simulink model "PID_Test"  (R2014b)
settings: Solver=ode14x  StartTime=0.0  StopTime=inf  FixedStep=0.2  RelTol=1e-3
undefined symbols (not defined in the file or in its folder): IsPositionTracked, IsSkeletonTracked, JointDepthIndices, JointImageIndices, JointTrackingState, JointWorldCoordinates, none, PositionDepthIndices, PositionImageIndices, PositionWorldCoordinates, SegmentationData, SkeletonTrackingID, videoinput
libraries: simulink x7, arduino_io_lib x2, visionsinks x2, visionstatistics x1, visiontextngfix x1, imaqlib x1, visiongeotforms x1
settings Model: Creator=mtsou_000  LastModifiedBy=mtsou_000

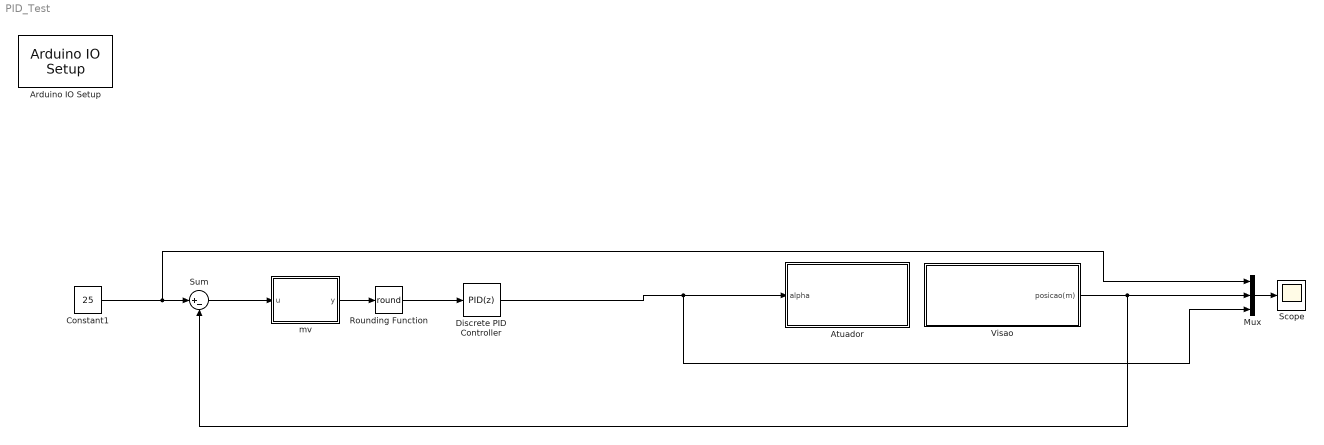
== system PID_Test ==
  Arduino IO Setup : arduino_io_lib/Arduino IO Setup  Priority=3  arduinoVar=Temporary arduino variable: Arduino1  workspaceVarName=a  comPort=COM8
  "Atuador " : Subsystem
  Constant1 : Constant  Value=25
  Discrete PID Controller : simulink/Continuous/PID Controller  Controller=PID  TimeDomain=Discrete-time  SampleTime=0.2  IntegratorMethod=Forward Euler  FilterMethod=Forward Euler  Form=Parallel  P=0.4  I=0.1  D=0.7  N=100  InitialConditionSource=internal  InitialConditionForIntegrator=0  InitialConditionForFilter=0  ExternalReset=none  LimitOutput=on  UpperSaturationLimit=30  LowerSaturationLimit=-30  LinearizeAsGain=off  AntiWindupMode=none  Kb=1  TrackingMode=off  Kt=1  PParamMin=[]  PParamMax=[]  IParamMin=[]  IParamMax=[]  DParamMin=[]  DParamMax=[]  NParamMin=[]  NParamMax=[]  KbParamMin=[]  KbParamMax=[]  KtParamMin=[]  KtParamMax=[]  POutMin=[]  POutMax=[]  IOutMin=[]  IOutMax=[]  DOutMin=[]  DOutMax=[]  NOutMin=[]  NOutMax=[]  KbOutMin=[]  KbOutMax=[]  KtOutMin=[]  KtOutMax=[]  IntegratorOutMin=[]  IntegratorOutMax=[]  FilterOutMin=[]  FilterOutMax=[]  SumOutMin=[]  SumOutMax=[]  SumI1OutMin=[]  SumI1OutMax=[]  SumI2OutMin=[]  SumI2OutMax=[]  SumI3OutMin=[]  SumI3OutMax=[]  SumDOutMin=[]  SumDOutMax=[]  SaturationOutMin=[]  SaturationOutMax=[]  IntegratorContinuousStateAttributes=''  IntegratorStateMustResolveToSignalObject=off  IntegratorRTWStateStorageClass=Auto  FilterContinuousStateAttributes=''  FilterStateMustResolveToSignalObject=off  FilterRTWStateStorageClass=Auto  DifferentiatorICPrevScaledInput=0  DifferentiatorOutMin=[]  DifferentiatorOutMax=[]  UseFilter=off
  Mux : Mux  Inputs=3
  Rounding Function : Rounding  Operator=round
  Scope : Scope
      settings: TickLabels=on  TimeRange=10  YMax=30
  Sum : Sum  Inputs=|+-
  Visao : Subsystem
  "mv " : MATLAB Function  TreatAsAtomicUnit=on
  wires:
  Sum/1 -> "mv "/1(u)
  "mv "/1(y) -> Rounding Function/1
  Mux/1 -> Scope/1
  Visao/1(posicao(m)) -> Mux/2, Sum/2
  Constant1/1 -> Mux/1, Sum/1
  Rounding Function/1 -> Discrete PID Controller/1
  Discrete PID Controller/1 -> Mux/3, "Atuador "/1(alpha)

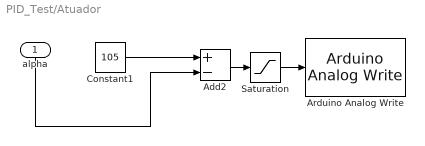
== system PID_Test/Atuador  ==
  alpha : Inport
  Add2 : Sum  Inputs=+-
  Arduino Analog Write : arduino_io_lib/Arduino Analog Write  arduinoVar=Temporary arduino variable: Arduino1  arduinoPin=3  T=0.2
  Constant1 : Constant  Value=105
  Saturation : Saturate  UpperLimit=120  LowerLimit=60
  wires:
  Add2/1 -> Saturation/1
  alpha/1 -> Add2/2
  Saturation/1 -> Arduino Analog Write/1
  Constant1/1 -> Add2/1

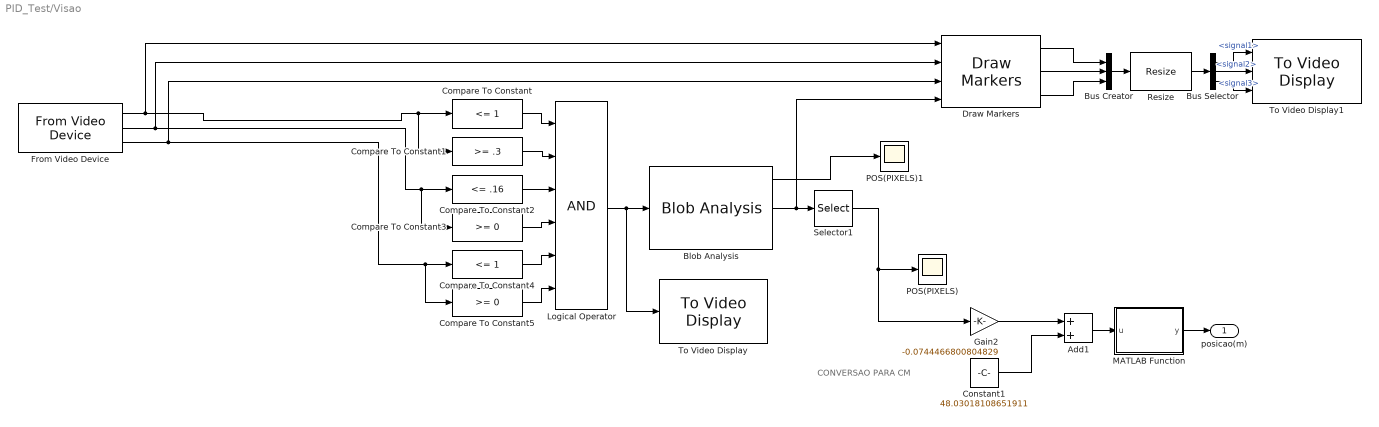
== system PID_Test/Visao ==
  note: CONVERSAO PARA CM
  Add1 : Sum
  Blob Analysis : visionstatistics/Blob Analysis  Tag=vipblks_row_conv  area=on  centroid=on  bBox=off  majorAxis=off  minorAxis=off  angle=off  eccentricity=off  equivDiameterSq=on  extent=off  perimeter=off  maxBlobs=1  warnIfNumBlobsExceeded=off  isCount=off  useMinArea=on  minArea=400  useMaxArea=off  maxArea=2200  excludeBorderBlob=off  outDT=double  isOutVarDim=off  isFill=on  fillValues=-1  conn=8  isLabel=off  outputMode=Binary point scaling  outputWordLength=32  outputFracLength=16  firstCoeffMode=Binary point scaling  firstCoeffWordLength=16  firstCoeffFracLength=14  secondCoeffMode=Binary point scaling  secondCoeffWordLength=32  secondCoeffFracLength=16  accumMode=Binary point scaling  accumWordLength=32  accumFracLength=0  prodOutputMode=Binary point scaling  prodOutputWordLength=32  prodOutputFracLength=16  roundingMode=Floor  overflowMode=off
  Bus Creator : BusCreator  Inputs=3
  Bus Selector : BusSelector
  Compare To Constant : simulink/Logic and Bit Operations/Compare To Constant  relop=<=  const=1  OutDataTypeStr=boolean
  Compare To Constant1 : simulink/Logic and Bit Operations/Compare To Constant  relop=>=  const=.3  OutDataTypeStr=boolean
  Compare To Constant2 : simulink/Logic and Bit Operations/Compare To Constant  relop=<=  const=.16  OutDataTypeStr=boolean
  Compare To Constant3 : simulink/Logic and Bit Operations/Compare To Constant  relop=>=  const=0  OutDataTypeStr=boolean
  Compare To Constant4 : simulink/Logic and Bit Operations/Compare To Constant  relop=<=  const=1  OutDataTypeStr=boolean
  Compare To Constant5 : simulink/Logic and Bit Operations/Compare To Constant  relop=>=  const=0  OutDataTypeStr=boolean
  Constant1 : Constant  Value=48.03018108651911
  Draw Markers : visiontextngfix/Draw Markers  shape=Circle  size=28  fill=on  fillClrSource=Specify via dialog  display=White  intensity=200  color=[200 255 100]  opacity=.5  viewport=Entire image  antialiasing=off  inType=Obsolete  imagePorts=Separate color signals  prodOutputMode=Binary point scaling  prodOutputWordLength=32  prodOutputFracLength=14  memoryMode=Specify word length  memoryWordLength=16  memoryFracLength=14  roundingMode=Floor  overflowMode=off
  From Video Device : imaqlib/From Video Device  DeviceMenu=winvideo 2 (Webcam 1200)  Device=winvideo 2 (Webcam 1200)  ObjConstructor=videoinput('winvideo', 2)  VideoFormatMenu=RGB24_640x480  VideoFormat=RGB24_640x480  VideoSource=input1  ROIPosition=[0 0 480 640]  EnableHWTrigger=off  TriggerConfiguration=none/none  SampleTime=0.2  OutputPortsMode=Separate color signals  DataType=single  CanDoHWTrigger=no  ReturnedColorSpace=rgb  BlockHandle=1921.0006  ROIWidth=640  ROIHeight=480  ROIColumn=0  ROIRow=0  EngXMLPath=C:\Program Files\MATLAB\R2014b\toolbox\imaq\imaq\private  DevXMLPath=C:\MATLAB\SupportPackages\R2014b\osgenericvideointerface\toolbox\imaq\supportpackages\genericvideo\adaptor\win64  EngLibPath=C:\Program Files\MATLAB\R2014b\toolbox\imaq\imaqblks\imaqmex\win64  ColorSpace=rgb  BayerSensorAlignment=grbg  AllMetadata=IsPositionTracked;IsSkeletonTracked;JointDepthIndices;JointImageIndices;JointTrackingState;JointWorldCoordinates;PositionDepthIndices;PositionImageIndices;PositionWorldCoordinates;SegmentationData;SkeletonTrackingID
  Gain2 : Gain  Gain=-0.0744466800804829
  Logical Operator : Logic  Inputs=6  AllPortsSameDT=off  OutDataTypeStr=boolean
  MATLAB Function : MATLAB Function  TreatAsAtomicUnit=on
  POS(PIXELS) : Scope
      settings: YMin=-2  YMax=0
  POS(PIXELS)1 : Scope
      settings: YMin=-500  YMax=2500  SaveName=ScopeData2
  Resize : visiongeotforms/Resize  specify=Number of output rows and columns  rfactor=[200 150]  outCols=25  outRows=25  outRowsCols=[300 400]  interp_method=Bilinear  antialias=on  useROI=off  roiFlag=off  prodOutputMode=Binary point scaling  prodOutputWordLength=32  prodOutputFracLength=10  roundingMode=Nearest  overflowMode=on
  Selector1 : Selector  NumberOfDimensions=2  InputPortWidth=2  IndexOptions=Index vector (dialog),Index vector (dialog)  Indices=1,1  OutputSizes=1,1
  To Video Display : visionsinks/To Video Display  inputType=Obsolete  imagePorts=One multidimensional signal  OutputDevice=On-screen video monitor  fullScreen=off  videoWindowX=684  videoWindowY=-1  saveWindowSize=off  videoWindowWidth=640  videoWindowHeight=480  dataOrg=Column-major  openAtMdlStart=on  isWindowOpen=on  inputColorFormat=RGB
  To Video Display1 : visionsinks/To Video Display  inputType=Obsolete  imagePorts=Separate color signals  OutputDevice=On-screen video monitor  fullScreen=off  videoWindowX=326  videoWindowY=238  saveWindowSize=off  videoWindowWidth=400  videoWindowHeight=300  dataOrg=Column-major  openAtMdlStart=on  isWindowOpen=off  inputColorFormat=RGB
  posicao(m) : Outport
  wires:
  Compare To Constant5/1 -> Logical Operator/6
  From Video Device/3 -> Draw Markers/3, Compare To Constant5/1, Compare To Constant4/1
  Compare To Constant/1 -> Logical Operator/1
  Logical Operator/1 -> To Video Display/1, Blob Analysis/1
  Compare To Constant1/1 -> Logical Operator/2
  From Video Device/2 -> Draw Markers/2, Compare To Constant2/1, Compare To Constant3/1
  Compare To Constant2/1 -> Logical Operator/3
  Compare To Constant4/1 -> Logical Operator/5
  Compare To Constant3/1 -> Logical Operator/4
  From Video Device/1 -> Draw Markers/1, Compare To Constant/1, Compare To Constant1/1
  Blob Analysis/2 -> Selector1/1, Draw Markers/4
  Bus Creator/1 -> Resize/1
  Resize/1 -> Bus Selector/1
  Bus Selector/1 -> To Video Display1/1  "<signal1>"
  Bus Selector/2 -> To Video Display1/2  "<signal2>"
  Bus Selector/3 -> To Video Display1/3  "<signal3>"
  Draw Markers/2 -> Bus Creator/2
  Draw Markers/1 -> Bus Creator/1
  Draw Markers/3 -> Bus Creator/3
  Selector1/1 -> Gain2/1, POS(PIXELS)/1
  Gain2/1 -> Add1/1
  Constant1/1 -> Add1/2
  Add1/1 -> MATLAB Function/1(u)
  Blob Analysis/1 -> POS(PIXELS)1/1
  MATLAB Function/1(y) -> posicao(m)/1

== matlab function PID_Test/mv  ==
  data: u input; y output
function y = fcn(u)

if (abs(u)<0.5)    
    u=0;
end

y=u;

== matlab function PID_Test/Visao/MATLAB Function ==
  data: u input; y output
function y = fcn(u)

persistent float ua;

if (isempty(ua))
    ua = 20;
end

if (abs(u-ua)>25)
    u = ua;
end

ua = u;
y=u;
